simulink model "Dc_motor_modeling_control"  (R2016a)
settings: Solver=ode23tb  StartTime=0.0  StopTime=10  MaxStep=1e-4  RelTol=1e-3
libraries: simulink x1, powerlib x1
settings Model: Creator=AT Once  LastModifiedBy=maxha

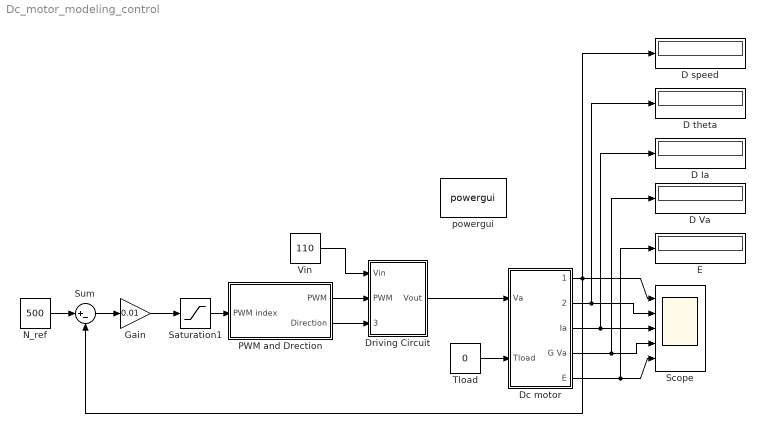
== system Dc_motor_modeling_control ==
  D Ia : Display
  D Va : Display
  D speed : Display
  D theta : Display
  Dc motor : Subsystem
  Driving Circuit : Subsystem
  E : Display
  Gain : Gain  Gain=0.01
  N_ref : Constant  Value=500
  PWM and Drection : Subsystem
  Saturation1 : Saturate  UpperLimit=+1  LowerLimit=-1
  Scope : Scope  NumInputPorts=5
  Sum : Sum  Inputs=|+-
  Tload : Constant  Value=0
  Vin : Constant  Value=110
  powergui : powerlib/powergui  Priority=1  SimulationMode=Continuous  SolverType=Tustin/Backward Euler (TBE)  SampleTime=50e-6  frequency=60  SPID=off  DisableSnubberDevices=off  DisableRonSwitches=off  DisableVfSwitches=off  SwTol=0  DisplayEquations=off  Interpol=off  ExternalGateDelay=off  methode=off  Ts=10  FunctionMessages=off  echomessages=off  HookPort=off  EnableUseOfTLC=off  x0status=blocks  frequencyindice=0  Pbase=100e6  ErrMax=1e-4  Iterations=50  UnitsV=kV  UnitsW=MW  buscounter=0  RestoreLinks=warning  ResistiveCurrentMeasurement=off  Frange=[0:2:500]  Ylog=off  Xlog=on  ShowGrid=off  save=off  variable=ZData  structure=0  ZoomFFT=off  StartTime=0.0  cycles=1  DisplayStyle=1  fundamental=60  FreqAxis=off  MaxFrequency=1000  frequencyindicesteady=1  RmsSteady=1  display=off
  wires:
  Tload/1 -> Dc motor/2(Tload)
  Dc motor/1(Speed) -> Sum/2, D speed/1, Scope/1
  Dc motor/2(Theta) -> D theta/1, Scope/2
  Dc motor/3(Ia) -> D Ia/1, Scope/3
  Dc motor/4(G Va) -> D Va/1, Scope/4
  Dc motor/5(E) -> E/1, Scope/5
  PWM and Drection/1(PWM) -> Driving Circuit/2(PWM)
  PWM and Drection/2(Direction) -> Driving Circuit/3(Direction)
  Vin/1 -> Driving Circuit/1(Vin)
  Driving Circuit/1(Vout) -> Dc motor/1(Va)
  Saturation1/1 -> PWM and Drection/1(PWM index)
  Gain/1 -> Saturation1/1
  N_ref/1 -> Sum/1
  Sum/1 -> Gain/1

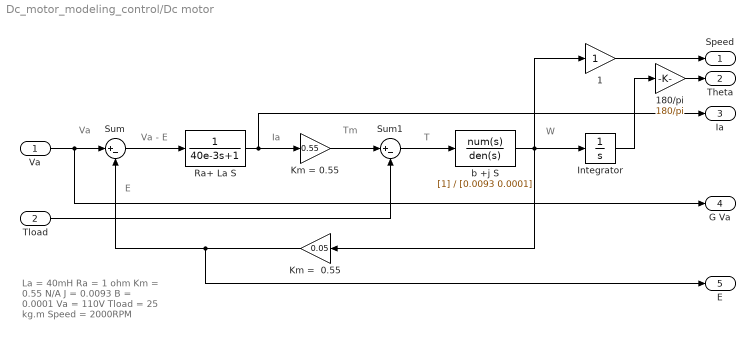
== system Dc_motor_modeling_control/Dc motor ==
  note: La = 40mH
      | Ra = 1 ohm
      | Km = 0.55 N/A
      | J = 0.0093
      | B = 0.0001
      | Va = 110V
      | Tload = 25 kg.m
      | Speed = 2000RPM
  note: E
  note: W
  note: T
  note: Tm
  note: Ia
  note: Va - E
  note: Va
  Va : Inport
  Tload : Inport  Port=2
  1 : Gain
  180/pi : Gain  Gain=180/pi
  Integrator : Integrator
  Km =  0.55 : Gain  Gain=0.05
  Km = 0.55 : Gain  Gain=0.55
  Ra+ La S : TransferFcn  Denominator=[40e-3 1]
  Sum : Sum  Inputs=|+-
  Sum1 : Sum  Inputs=|+-
  b +j S : TransferFcn  Denominator=[0.0093 0.0001]
  Speed : Outport
  Theta : Outport  Port=2
  Ia : Outport  Port=3
  G Va : Outport  Port=4
  E : Outport  Port=5
  wires:
  Va/1 -> G Va/1, Sum/1
  Ra+ La S/1 -> Ia/1, Km = 0.55/1
  Tload/1 -> Sum1/2
  b +j S/1 -> 1/1, Km =  0.55/1, Integrator/1
  Sum1/1 -> b +j S/1
  Km = 0.55/1 -> Sum1/1
  Km =  0.55/1 -> E/1, Sum/2
  Sum/1 -> Ra+ La S/1
  1/1 -> Speed/1
  180/pi/1 -> Theta/1
  Integrator/1 -> 180/pi/1

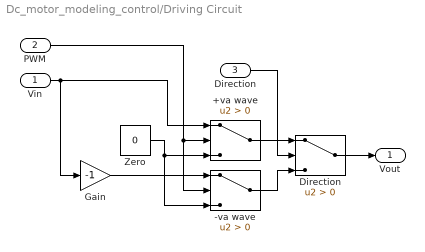
== system Dc_motor_modeling_control/Driving Circuit ==
  Vin : Inport
  PWM : Inport  Port=2
  Direction : Inport  Port=3
  +va wave : Switch  Criteria=u2 > Threshold
  -va wave : Switch  Criteria=u2 > Threshold
  "Direction " : Switch  Criteria=u2 > Threshold
  Gain : Gain  Gain=-1
  Zero : Constant  Value=0
  Vout : Outport
  wires:
  +va wave/1 -> "Direction "/1
  Zero/1 -> +va wave/3, -va wave/3
  -va wave/1 -> "Direction "/3
  Direction/1 -> "Direction "/2
  "Direction "/1 -> Vout/1
  Gain/1 -> -va wave/1
  PWM/1 -> +va wave/2, -va wave/2
  Vin/1 -> +va wave/1, Gain/1

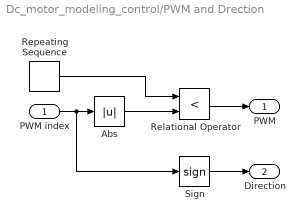
== system Dc_motor_modeling_control/PWM and Drection ==
  PWM index : Inport
  Abs : Abs
  Relational Operator : RelationalOperator  Operator=<  OutDataTypeStr=boolean
  Repeating Sequence : simulink/Sources/Repeating Sequence  rep_seq_t=[0 1 1.000000001 2]*1e-3  rep_seq_y=[1 0 1 0]
  Sign : Signum
  PWM : Outport
  Direction : Outport  Port=2
  wires:
  Repeating Sequence/1 -> Relational Operator/1
  Abs/1 -> Relational Operator/2
  Sign/1 -> Direction/1
  Relational Operator/1 -> PWM/1
  PWM index/1 -> Sign/1, Abs/1
